simulink model "STEVE_Simulation"  (R2024b)
settings: Solver=ode8  StartTime=0.0  StopTime=Sim.Time  FixedStep=Sim.Timestep  RelTol=1e-3  EnableMultiTasking=on
values from neighbouring files (symbols this model uses):
  AeroData = CombinedAeroData    [initialize_sim_parameters.m]
  m = 1277.9    [LQR_Controller_Design.m]    (also in controlability_analysis.m = params.mass(i); lqr_gain_scedule.m = interp_data.mass(i); matlab.mat = 974)
  q = 0.5 * rho * V^2    (= 29036.16)    [LQR_Controller_Design.m]    (also in matlab.mat = 2919.616)
  Ref_Area = RocketAeroPhysical.Reference_Area    [initialize_sim_parameters.m]
undefined symbols (not defined in the file or in its folder): Actuators, Earth, F, Initial, Light, MIL, PrelookupData, rocket_length, RocketAeroPhysical, s, ThrustLookupData, timeStep, WGS84
libraries: simulink x6, simulink_extras x4, aerolibwind2 x4, aerolibtransform2 x3, aerolibasang x3, aerolibconvert2 x2, aerolibnav x2, aerolibactuator x2, aerolibatmos2 x1, dspsrcs4 x1, mspfiltlib x1, sharedtransform x1
(part 2 of 2)

== matlab function STEVE_Simulation/STeVe System Model/Vehicle Dynamics/RocketEngineActuators/MATLAB Function ==
  data: delta_S input; theta_nozzle_rad output
function theta_nozzle_rad = linkage_to_nozzle_angle(delta_S)
% Calculates nozzle angle deflection based on linear actuator displacement (delta_S).
% Assumes delta_S is the change in length from the initial actuator length S0.
% theta_nozzle_rad is the CHANGE in the angle between linkage arms from their initial configuration.
% Input delta_S is expected in meters.
% Output theta_nozzle_rad is in radians.

%#codegen % Required for Simulink code generation

% Linkage parameters (constants)
l = 0.173086;   % m (First arm length)
r = 0.187926;   % m (Second arm length)
S0 = 0.221779;  % m (Initial actuator length when theta_nozzle_rad is defined as 0)

% --- Calculate the initial internal angle based on S0, l, and r ---
% This is the angle between arms l and r when delta_S = 0.
% cos(initial_internal_angle) = (l^2 + r^2 - S0^2) / (2 * l * r)
cos_arg_initial = (l^2 + r^2 - S0^2) / (2 * l * r);

% Clamp for safety, though with consistent S0, l, r, it should be valid
if cos_arg_initial > 1.0
    cos_arg_initial = 1.0;
elseif cos_arg_initial < -1.0
    cos_arg_initial = -1.0;
end
initial_internal_angle_rad = acos(cos_arg_initial);
% --------------------------------------------------------------------

% Calculate current total actuator length
S_current = S0 + delta_S;

% Calculate the argument for acos for the CURRENT internal angle
% cos(current_internal_angle) = (l^2 + r^2 - S_current^2) / (2 * l * r)
cos_arg_current = (l^2 + r^2 - S_current^2) / (2 * l * r);

% Clamp cos_arg_current to the valid range [-1, 1]
if cos_arg_current > 1.0
    cos_arg_current = 1.0;
elseif cos_arg_current < -1.0
    cos_arg_current = -1.0;
end

% Calculate current internal angle between arms l and r
current_internal_angle_rad = acos(cos_arg_current); % Result is in radians

% Calculate theta_nozzle_rad as the CHANGE from the initial internal angle
theta_nozzle_rad = current_internal_angle_rad - initial_internal_angle_rad;

% --- Optional: Map this change in internal angle to actual nozzle orientation ---
% If the nozzle's zero position (theta_nozzle_rad = 0) corresponds to a specific
% absolute orientation (e.g., aligned with rocket body), and 'alpha_deg' from your
% original code represented some offset or component of the initial nozzle orientation,
% you might need an additional step.
% For example, if alpha_deg was an offset:
% nozzle_absolute_angle_rad = theta_nozzle_rad + (alpha_deg_from_original_code * pi/180);
% But based on your problem description, the current theta_nozzle_rad (as a change)
% is likely what's needed if delta_S=0 should give theta_nozzle_rad=0.
end

== matlab function STEVE_Simulation/STeVe System Model/Vehicle Dynamics/Aerodynamics/Force Calculations/Pitch Moment Damping1 ==
  data: Lcg input; Deq input; Lref input; M_damp output; Lfuselage input; Aref input; q_pitch input; Cmq_fuselage output; V input; q_bar input
function [M_damp, Cmq_fuselage] = DampingMoment(Lcg, Deq, Lref, Lfuselage, Aref, q_pitch, V, q_bar)
% Calculates Cmq_fuselage based on Eq. 5-51 [1] and the resulting pitch damping moment M_damp.
% WARNING: Eq. 5-51 defines Cmq with a (q/V)^2 term. Using this Cmq in the
% standard linear moment formula M_damp = q_bar*Aref*Lref*Cmq*(q*Lref/V)
% results in a damping moment proportional to q_pitch^3. Verify this is intended.
%
% Inputs:
%   Deq       : Equivalent diameter of the fuselage [length]
%   Lcg       : Longitudinal CG position from fuselage start [length]
%   Lfuselage : Total length of the fuselage [length] (Assumed = l in Eq. 5-51)
%   Aref      : Reference area [length^2] (Assumed = A in Eq. 5-51)
%   Lref      : Reference length for moment calculation [length]
%   q_pitch   : Pitch rate [rad/s] (q in Eq. 5-51)
%   V         : Airspeed [length/s] (va in Eq. 5-51)
%   q_bar     : Dynamic pressure [Force/Area]
%
% Outputs:
%   M_damp       : Pitch damping moment [Force*Length]
%   Cmq_fuselage : Fuselage pitch damping coefficient from Eq. 5-51 (non-dimensional)

% --- Input Validation (Basic) ---
if V < 0 || Aref <= 0 || Lfuselage <= 0 || Deq < 0 || Lref <= 0 || q_bar < 0
    error('Inputs V, Aref, Lfuselage, Deq, Lref, q_bar must be non-negative/positive as appropriate.');
end
% Note: More extensive validation could be added (e.g., Lcg range).

% --- Step 1: Calculate Cmq_fuselage using Eq. 5-51 ---

% Geometric term numerator
numerator_geom = 1.1 * Deq * (Lcg^4 + (Lfuselage - Lcg)^4);

% Geometric term denominator (Assuming l = Lfuselage, A = Aref)
denominator_geom = 4 * Lfuselage * Aref;

% Non-dimensional pitch rate squared term (q/V)^2
% Handle potential division by zero if V is very small or zero
if abs(V) < eps % Check if V is close to zero
    nd_pitch_rate_sq = 0;
    if abs(q_pitch) > eps
        % Optional: Use coder.extrinsic('warning') for warnings in generated code
        % warning('SimBlk:VnearZero', 'Airspeed V is near zero, but pitch rate q is non-zero. Setting (q/V)^2 term to 0.');
    end
else
    nd_pitch_rate_sq = (q_pitch / V)^2;
end

% Combine terms for Cmq_fuselage
if abs(denominator_geom) < eps
     error('Denominator (4 * Lfuselage * Aref) is near zero.');
end
Cmq_fuselage = (numerator_geom / denominator_geom) * nd_pitch_rate_sq;

% --- Step 2: Calculate M_damp using standard formula ---

% Reduced angular rate term (q*Lref/V)
% Handle potential division by zero if V is very small or zero
if abs(V) < eps % Check if V is close to zero
    reduced_rate_term = 0;
     if abs(q_pitch) > eps
        % Optional: Use coder.extrinsic('warning')
        % warning('SimBlk:VnearZero', 'Airspeed V is near zero, but pitch rate q is non-zero. Setting reduced rate term to 0.');
     end
else
    reduced_rate_term = (q_pitch * Lref) / V;
end

% Calculate damping moment
M_damp = q_bar * Aref * Lref * Cmq_fuselage * reduced_rate_term;

end

% [1] Reference: Image containing Equation 5-51 provided in the search results.
